simulink model "PfLoad"  (R2022a)
settings: Solver=ode14x  StartTime=0  StopTime=Sim.tend  FixedStep=0.000125  RelTol=4e-4
model workspace (MAT data in the model file):
  nr_load = Simulink.Parameter
  nr_load.Value = 2
  nr_load.DataType = 'int8'
  nr_load.Complexity = 'real'
  nr_load.Dimensions = [1 1]
values from neighbouring files (symbols this model uses):
  ControlSampleTime = 1/8000    (= 0.000125)    [sim3run_390.m]
  FB_area1_downlim = 49.5    [prm3var_390.m]
  FB_area1_uplim = 49.8    [prm3var_390.m]
  FB_area2_downlim = 49.2    [prm3var_390.m]
  FB_area2_uplim = 49.5    [prm3var_390.m]
  TVint = 0.05    [prm3var_390.m]
undefined symbols (not defined in the file or in its folder): DiscIntNeverNeededParam, General, parameterset, prm_load, pu_vsm, UFLS
libraries: simulink x2
settings Model: ParameterArgumentNames=nr_load  Creator=e2n052  LastModifiedBy=uk062294
settings DataIOCC: SaveOutput=off  SaveTime=off  ReturnWorkspaceOutputs=off
settings DebuggingCC: UnconnectedInputMsg=warning  UnconnectedOutputMsg=warning  UnconnectedLineMsg=warning  ArithmeticOperatorsInVariantConditions=warning
settings SFSimCC: SimUseLocalCustomCode=off  CustomCodeUndefinedFunction=UseInterfaceOnly
settings RTWCC: RTWUseLocalCustomCode=off  DLArmComputeVersion=19.05

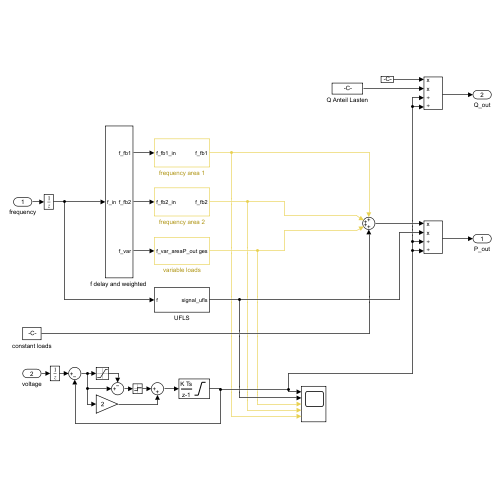
[thumbnail: Simulink's stored preview of the top-level diagram]
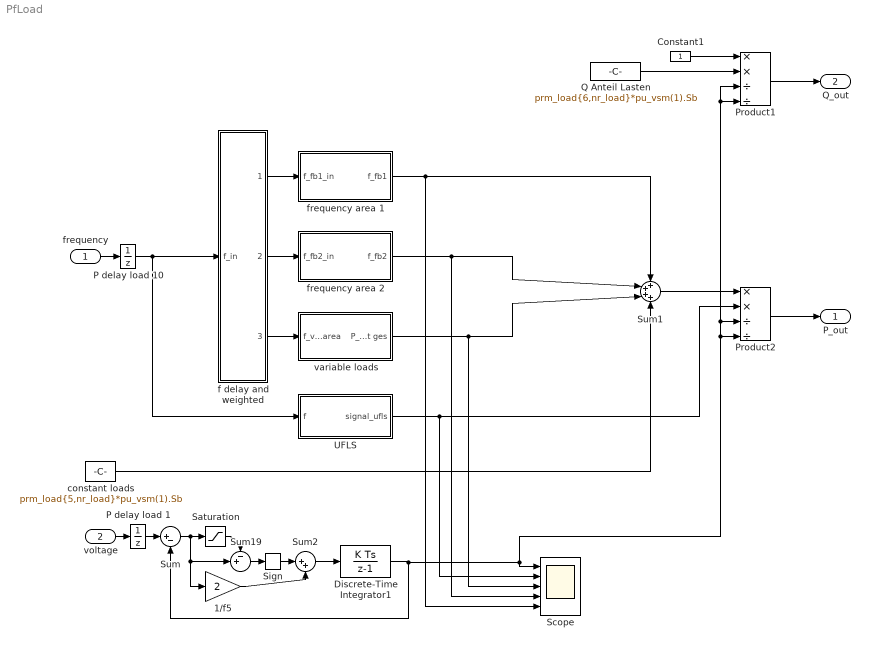
== system PfLoad ==
  frequency : Inport
  voltage : Inport  Port=2
  1/f5 : Gain  Gain=2
  Constant1 : Constant
  Discrete-Time Integrator1 : DiscreteIntegrator  gainval=1/TVint  InitialCondition=1  SampleTime=-1  LimitOutput=on  UpperSaturationLimit=1.15  LowerSaturationLimit=0.85  ICPrevOutput=DiscIntNeverNeededParam  ICPrevScaledInput=DiscIntNeverNeededParam
  P delay load 1 : UnitDelay  InitialCondition=General.Vnreg  SampleTime=-1  HasFrameUpgradeWarning=on
  P delay load 10 : UnitDelay  InitialCondition=General.fn  SampleTime=-1  HasFrameUpgradeWarning=on
  Product1 : Product  Inputs=**//
  Product2 : Product  Inputs=**//
  Q Anteil Lasten : Constant  Value=prm_load{6,nr_load}*pu_vsm(1).Sb
  Saturation : Saturate  UpperLimit=0.03  LowerLimit=-0.03
  Scope : Scope  NumInputPorts=5
  Sign : Signum
  Sum : Sum  Inputs=|+-
  Sum1 : Sum  Inputs=++++
  Sum19 : Sum  Inputs=-+|
  Sum2 : Sum  Inputs=|++
  UFLS : Subsystem
  constant loads : Constant  Value=prm_load{5,nr_load}*pu_vsm(1).Sb
  "f delay and weighted " : Subsystem
  frequency area 1 : Subsystem
  frequency area 2 : Subsystem
  variable loads : Subsystem
  P_out : Outport  OutDataTypeStr=double  PortDimensions=1
  Q_out : Outport  Port=2  OutDataTypeStr=double  PortDimensions=1
  wires:
  frequency area 1/1(f_fb1) -> Scope/5, Sum1/1
  frequency area 2/1(f_fb2) -> Scope/4, Sum1/2
  variable loads/1(P_out ges) -> Scope/3, Sum1/3
  constant loads/1 -> Sum1/4
  Sum1/1 -> Product2/1
  Constant1/1 -> Product1/1
  Q Anteil Lasten/1 -> Product1/2
  frequency/1 -> P delay load 10/1
  UFLS/1(signal_ufls) -> Scope/2, Product2/2
  "f delay and weighted "/1(f_fb1) -> frequency area 1/1(f_fb1_in)
  "f delay and weighted "/2(f_fb2) -> frequency area 2/1(f_fb2_in)
  "f delay and weighted "/3(f_var) -> variable loads/1(f_var_area)
  Sum/1 -> Sum19/2, 1/f5/1, Saturation/1
  Discrete-Time Integrator1/1 -> Sum/2, Scope/1, Product2/4, Product2/3, Product1/4, Product1/3
  Product1/1 -> Q_out/1
  Product2/1 -> P_out/1
  P delay load 10/1 -> "f delay and weighted "/1(f_in), UFLS/1(f)
  voltage/1 -> P delay load 1/1
  P delay load 1/1 -> Sum/1
  Saturation/1 -> Sum19/1
  Sign/1 -> Sum2/1
  Sum19/1 -> Sign/1
  Sum2/1 -> Discrete-Time Integrator1/1
  1/f5/1 -> Sum2/2

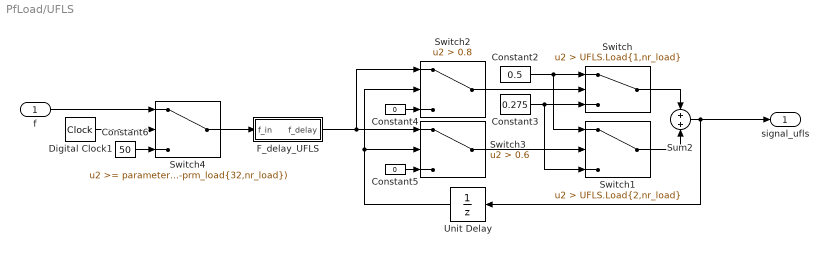
== system PfLoad/UFLS ==
  f : Inport
  Constant2 : Constant  Value=0.5
  Constant3 : Constant  Value=0.275
  Constant4 : Constant  Value=0
  Constant5 : Constant  Value=0
  Constant6 : Constant  Value=50
  Digital Clock1 : DigitalClock  SampleTime=ControlSampleTime
  F_delay_UFLS : Subsystem
  Sum2 : Sum  Inputs=+|+
  Switch : Switch  Criteria=u2 > Threshold  Threshold=UFLS.Load{1,nr_load}  SaturateOnIntegerOverflow=off  InputSameDT=off
  Switch1 : Switch  Criteria=u2 > Threshold  Threshold=UFLS.Load{2,nr_load}  SaturateOnIntegerOverflow=off  InputSameDT=off
  Switch2 : Switch  Criteria=u2 > Threshold  Threshold=0.8  SaturateOnIntegerOverflow=off  InputSameDT=off
  Switch3 : Switch  Criteria=u2 > Threshold  Threshold=0.6  SaturateOnIntegerOverflow=off  InputSameDT=off
  Switch4 : Switch  Threshold=parameterset.Event.IslandingTime-0.1+9e9*(1-prm_load{32,nr_load})  SaturateOnIntegerOverflow=off  InputSameDT=off
  Unit Delay : UnitDelay  InitialCondition=50  SampleTime=-1  HasFrameUpgradeWarning=on
  signal_ufls : Outport
  wires:
  Switch/1 -> Sum2/1
  Sum2/1 -> signal_ufls/1, Unit Delay/1
  Constant4/1 -> Switch2/3
  Constant3/1 -> Switch1/3, Switch/3
  Constant6/1 -> Switch4/3
  f/1 -> Switch4/1
  Switch3/1 -> Switch1/2
  Constant5/1 -> Switch3/3
  Unit Delay/1 -> Switch3/2, Switch2/2
  Constant2/1 -> Switch1/1, Switch/1
  Switch2/1 -> Switch/2
  Switch1/1 -> Sum2/2
  Switch4/1 -> F_delay_UFLS/1(f_in)
  F_delay_UFLS/1(f_delay) -> Switch2/1, Switch3/1
  Digital Clock1/1 -> Switch4/2

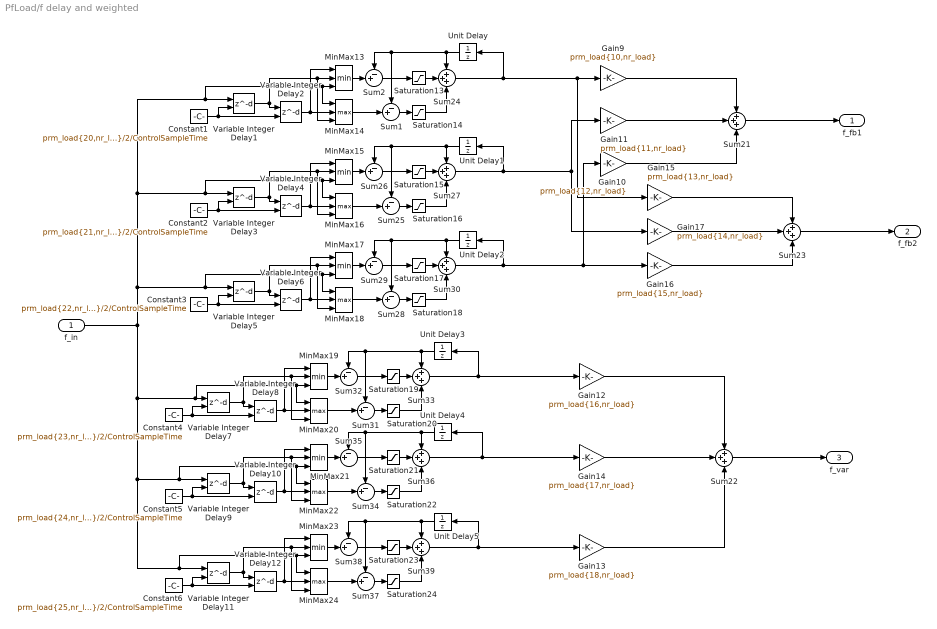
== system PfLoad/f delay and weighted  ==
  f_in : Inport
  Constant1 : Constant  Value=prm_load{20,nr_load}/2/ControlSampleTime
  Constant2 : Constant  Value=prm_load{21,nr_load}/2/ControlSampleTime
  Constant3 : Constant  Value=prm_load{22,nr_load}/2/ControlSampleTime
  Constant4 : Constant  Value=prm_load{23,nr_load}/2/ControlSampleTime
  Constant5 : Constant  Value=prm_load{24,nr_load}/2/ControlSampleTime
  Constant6 : Constant  Value=prm_load{25,nr_load}/2/ControlSampleTime
  Gain10 : Gain  Gain=prm_load{12,nr_load}
  Gain11 : Gain  Gain=prm_load{11,nr_load}
  Gain12 : Gain  Gain=prm_load{16,nr_load}
  Gain13 : Gain  Gain=prm_load{18,nr_load}
  Gain14 : Gain  Gain=prm_load{17,nr_load}
  Gain15 : Gain  Gain=prm_load{13,nr_load}
  Gain16 : Gain  Gain=prm_load{15,nr_load}
  Gain17 : Gain  Gain=prm_load{14,nr_load}
  Gain9 : Gain  Gain=prm_load{10,nr_load}
  MinMax{13,15,17,19,21,23} (6 alike) : MinMax  Inputs=3
  MinMax{14,16,18,20,22,24} (6 alike) : MinMax  Function=max  Inputs=3
  Saturation{13,15,17,19,21,23} (6 alike) : Saturate  UpperLimit=inf  LowerLimit=0
  Saturation{14,16,18,20,22,24} (6 alike) : Saturate  UpperLimit=0  LowerLimit=-inf
  Sum{1..2,25..26,28..29,31..32,34..35,37..38} (12 alike) : Sum  Inputs=-+|
  Sum{21..24,27,30,33,36,39} (9 alike) : Sum  Inputs=+++
  Unit Delay{,1..5} (6 alike) : UnitDelay  InitialCondition=General.fn  SampleTime=-1  HasFrameUpgradeWarning=on
  Variable Integer Delay{1..12} (12 alike) : Delay  DelayLengthSource=Input port  DelayLength=prm_load{21,nr_load}/2/ControlSampleTime  DelayLengthUpperLimit=5000
      settings: InputPortMap=u0,p1
  f_fb1 : Outport
  f_fb2 : Outport  Port=2
  f_var : Outport  Port=3
  wires:
  Gain14/1 -> Sum22/2
  Gain11/1 -> Sum21/2
  Gain10/1 -> Sum21/3
  Gain17/1 -> Sum23/2
  Gain15/1 -> Sum23/1
  Sum22/1 -> f_var/1
  Sum21/1 -> f_fb1/1
  Sum23/1 -> f_fb2/1
  Gain13/1 -> Sum22/3
  Gain16/1 -> Sum23/3
  Gain9/1 -> Sum21/1
  Gain12/1 -> Sum22/1
  Saturation14/1 -> Sum24/3
  Sum24/1 -> Unit Delay/1, Gain9/1, Gain15/1
  Sum1/1 -> Saturation14/1
  Unit Delay/1 -> Sum24/1, Sum2/1, Sum1/1
  Variable Integer Delay2/1 -> MinMax13/1, MinMax14/2
  Variable Integer Delay1/1 -> Variable Integer Delay2/1, MinMax14/3, MinMax13/2
  Constant1/1 -> Variable Integer Delay2/2, Variable Integer Delay1/2
  MinMax13/1 -> Sum2/2
  Sum2/1 -> Saturation13/1
  MinMax14/1 -> Sum1/2
  Saturation13/1 -> Sum24/2
  Saturation16/1 -> Sum27/3
  Sum25/1 -> Saturation16/1
  Unit Delay1/1 -> Sum27/1, Sum26/1, Sum25/1
  Variable Integer Delay4/1 -> MinMax15/1, MinMax16/2
  Variable Integer Delay3/1 -> Variable Integer Delay4/1, MinMax16/3, MinMax15/2
  Constant2/1 -> Variable Integer Delay4/2, Variable Integer Delay3/2
  MinMax15/1 -> Sum26/2
  Sum26/1 -> Saturation15/1
  MinMax16/1 -> Sum25/2
  Saturation15/1 -> Sum27/2
  Saturation18/1 -> Sum30/3
  Sum30/1 -> Unit Delay2/1, Gain10/1, Gain16/1
  Sum28/1 -> Saturation18/1
  Unit Delay2/1 -> Sum30/1, Sum29/1, Sum28/1
  Variable Integer Delay6/1 -> MinMax17/1, MinMax18/2
  Variable Integer Delay5/1 -> Variable Integer Delay6/1, MinMax18/3, MinMax17/2
  Constant3/1 -> Variable Integer Delay6/2, Variable Integer Delay5/2
  MinMax17/1 -> Sum29/2
  Sum29/1 -> Saturation17/1
  MinMax18/1 -> Sum28/2
  Saturation17/1 -> Sum30/2
  Saturation20/1 -> Sum33/3
  Sum31/1 -> Saturation20/1
  Unit Delay3/1 -> Sum33/1, Sum32/1, Sum31/1
  Variable Integer Delay8/1 -> MinMax19/1, MinMax20/2
  Variable Integer Delay7/1 -> Variable Integer Delay8/1, MinMax20/3, MinMax19/2
  Constant4/1 -> Variable Integer Delay8/2, Variable Integer Delay7/2
  MinMax19/1 -> Sum32/2
  Sum32/1 -> Saturation19/1
  MinMax20/1 -> Sum31/2
  Saturation19/1 -> Sum33/2
  Saturation22/1 -> Sum36/3
  Sum34/1 -> Saturation22/1
  Unit Delay4/1 -> Sum35/1, Sum34/1, Sum36/1
  Variable Integer Delay10/1 -> MinMax21/1, MinMax22/2
  Variable Integer Delay9/1 -> Variable Integer Delay10/1, MinMax22/3, MinMax21/2
  Constant5/1 -> Variable Integer Delay10/2, Variable Integer Delay9/2
  MinMax21/1 -> Sum35/2
  Sum35/1 -> Saturation21/1
  MinMax22/1 -> Sum34/2
  Saturation21/1 -> Sum36/2
  Saturation24/1 -> Sum39/3
  Sum37/1 -> Saturation24/1
  Unit Delay5/1 -> Sum39/1, Sum38/1, Sum37/1
  Variable Integer Delay12/1 -> MinMax23/1, MinMax24/2
  Variable Integer Delay11/1 -> Variable Integer Delay12/1, MinMax24/3, MinMax23/2
  f_in/1 -> MinMax24/1, MinMax23/3, Variable Integer Delay11/1, MinMax22/1, MinMax21/3, Variable Integer Delay9/1, MinMax20/1, MinMax19/3, Variable Integer Delay7/1, MinMax14/1, MinMax13/3, Variable Integer Delay1/1, MinMax16/1, MinMax15/3, Variable Integer Delay3/1, MinMax18/1, MinMax17/3, Variable Integer Delay5/1
  Constant6/1 -> Variable Integer Delay12/2, Variable Integer Delay11/2
  MinMax23/1 -> Sum38/2
  Sum38/1 -> Saturation23/1
  MinMax24/1 -> Sum37/2
  Saturation23/1 -> Sum39/2
  Sum27/1 -> Unit Delay1/1, Gain11/1, Gain17/1
  Sum33/1 -> Unit Delay3/1, Gain12/1
  Sum36/1 -> Unit Delay4/1, Gain14/1
  Sum39/1 -> Unit Delay5/1, Gain13/1

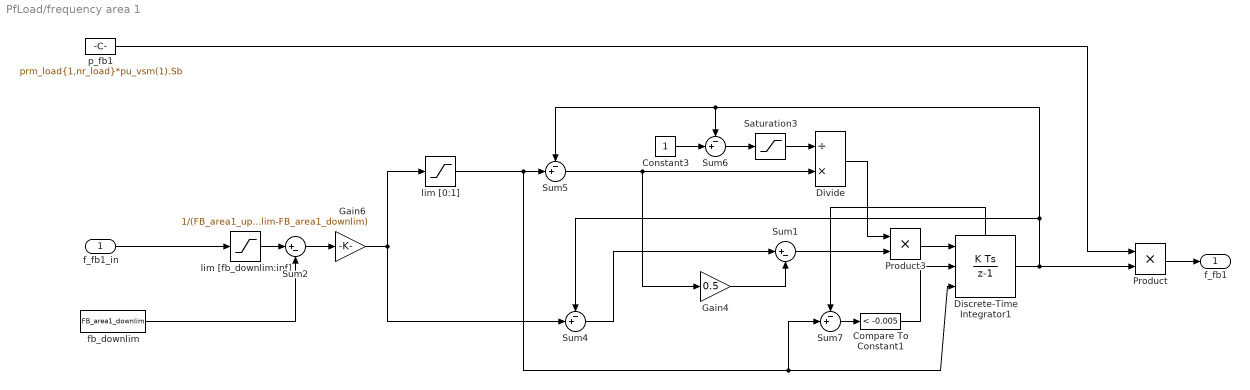
== system PfLoad/frequency area 1 ==
  f_fb1_in : Inport
  Compare To Constant1 : simulink/Logic and Bit Operations/Compare To Constant  relop=<  const=-0.005  OutDataTypeStr=boolean
  Constant3 : Constant
  Discrete-Time Integrator1 : DiscreteIntegrator  ExternalReset=level  InitialConditionSource=external  SampleTime=ControlSampleTime  LimitOutput=on  UpperSaturationLimit=1  LowerSaturationLimit=0  ShowStatePort=on  ICPrevOutput=DiscIntNeverNeededParam  ICPrevScaledInput=DiscIntNeverNeededParam
  Divide : Product  Inputs=/*
  Gain4 : Gain  Gain=0.5
  Gain6 : Gain  Gain=1/(FB_area1_uplim-FB_area1_downlim)
  Product : Product
  Product3 : Product
  Saturation3 : Saturate  UpperLimit=inf  LowerLimit=1e-6
  Sum1 : Sum  Inputs=|+-
  Sum2 : Sum  Inputs=|+-
  Sum{4..7} (4 alike) : Sum  Inputs=-+|
  fb_downlim : Constant  Value=FB_area1_downlim
  lim [0:1] : Saturate  UpperLimit=1  LowerLimit=0
  lim [fb_downlim:inf] : Saturate  UpperLimit=inf  LowerLimit=FB_area1_downlim
  p_fb1 : Constant  Value=prm_load{1,nr_load}*pu_vsm(1).Sb
  f_fb1 : Outport
  wires:
  Discrete-Time Integrator1/1 -> Sum5/1, Sum6/1, Sum4/1, Product/2
  Discrete-Time Integrator1/State -> Sum7/1
  Sum7/1 -> Compare To Constant1/1
  fb_downlim/1 -> Sum2/2
  f_fb1_in/1 -> lim [fb_downlim:inf]/1
  Compare To Constant1/1 -> Discrete-Time Integrator1/2
  Saturation3/1 -> Divide/1
  Divide/1 -> Product3/1
  Constant3/1 -> Sum6/2
  Gain6/1 -> Sum4/2, lim [0:1]/1
  Sum2/1 -> Gain6/1
  lim [fb_downlim:inf]/1 -> Sum2/1
  Sum4/1 -> Sum1/1
  Sum6/1 -> Saturation3/1
  Product3/1 -> Discrete-Time Integrator1/1
  Gain4/1 -> Sum1/2
  Sum5/1 -> Gain4/1, Divide/2
  Sum1/1 -> Product3/2
  lim [0:1]/1 -> Sum7/2, Discrete-Time Integrator1/3, Sum5/2
  Product/1 -> f_fb1/1
  p_fb1/1 -> Product/1

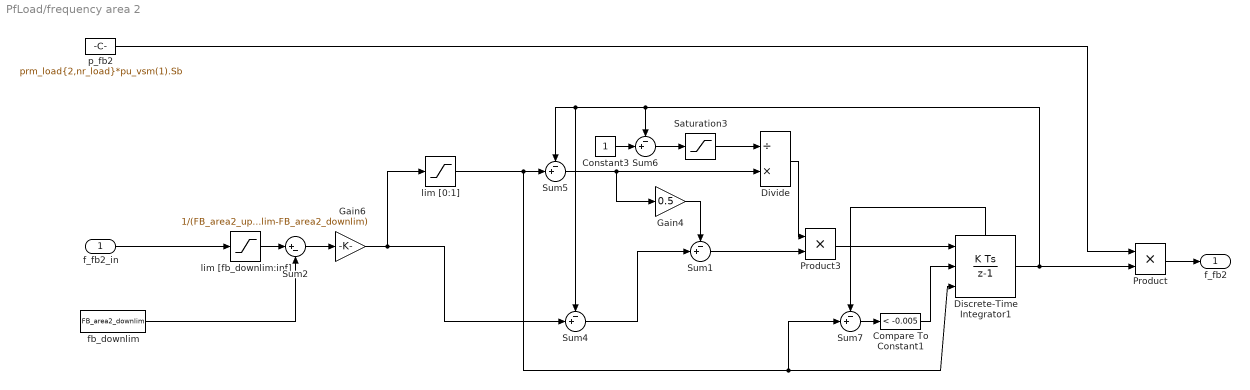
== system PfLoad/frequency area 2 ==
  f_fb2_in : Inport
  Compare To Constant1 : simulink/Logic and Bit Operations/Compare To Constant  relop=<  const=-0.005  OutDataTypeStr=boolean
  Constant3 : Constant
  Discrete-Time Integrator1 : DiscreteIntegrator  ExternalReset=level  InitialConditionSource=external  SampleTime=ControlSampleTime  LimitOutput=on  UpperSaturationLimit=1  LowerSaturationLimit=0  ShowStatePort=on  ICPrevOutput=DiscIntNeverNeededParam  ICPrevScaledInput=DiscIntNeverNeededParam
  Divide : Product  Inputs=/*
  Gain4 : Gain  Gain=0.5
  Gain6 : Gain  Gain=1/(FB_area2_uplim-FB_area2_downlim)
  Product : Product
  Product3 : Product
  Saturation3 : Saturate  UpperLimit=inf  LowerLimit=1e-6
  Sum{1,4..7} (5 alike) : Sum  Inputs=-+|
  Sum2 : Sum  Inputs=|+-
  fb_downlim : Constant  Value=FB_area2_downlim
  lim [0:1] : Saturate  UpperLimit=1  LowerLimit=0
  lim [fb_downlim:inf] : Saturate  UpperLimit=inf  LowerLimit=FB_area2_downlim
  p_fb2 : Constant  Value=prm_load{2,nr_load}*pu_vsm(1).Sb
  f_fb2 : Outport
  wires:
  Discrete-Time Integrator1/1 -> Sum4/1, Sum5/1, Sum6/1, Product/2
  Discrete-Time Integrator1/State -> Sum7/1
  Sum7/1 -> Compare To Constant1/1
  fb_downlim/1 -> Sum2/2
  f_fb2_in/1 -> lim [fb_downlim:inf]/1
  Compare To Constant1/1 -> Discrete-Time Integrator1/2
  Saturation3/1 -> Divide/1
  Divide/1 -> Product3/1
  Constant3/1 -> Sum6/2
  Gain6/1 -> Sum4/2, lim [0:1]/1
  Sum2/1 -> Gain6/1
  lim [fb_downlim:inf]/1 -> Sum2/1
  Sum4/1 -> Sum1/2
  Sum6/1 -> Saturation3/1
  Product3/1 -> Discrete-Time Integrator1/1
  Gain4/1 -> Sum1/1
  Sum5/1 -> Divide/2, Gain4/1
  Sum1/1 -> Product3/2
  lim [0:1]/1 -> Sum7/2, Discrete-Time Integrator1/3, Sum5/2
  Product/1 -> f_fb2/1
  p_fb2/1 -> Product/1

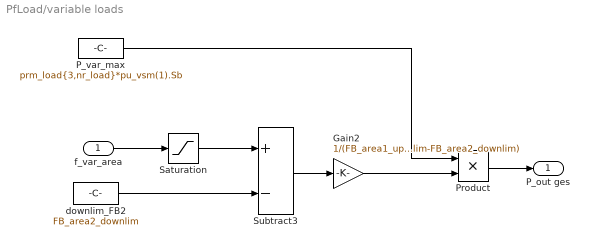
== system PfLoad/variable loads ==
  f_var_area : Inport
  Gain2 : Gain  Gain=1/(FB_area1_uplim-FB_area2_downlim)
  P_var_max : Constant  Value=prm_load{3,nr_load}*pu_vsm(1).Sb
  Product : Product
  Saturation : Saturate  UpperLimit=FB_area1_uplim  LowerLimit=FB_area2_downlim
  Subtract3 : Sum  Inputs=+-
  downlim_FB2 : Constant  Value=FB_area2_downlim
  P_out ges : Outport
  wires:
  Gain2/1 -> Product/2
  Subtract3/1 -> Gain2/1
  downlim_FB2/1 -> Subtract3/2
  f_var_area/1 -> Saturation/1
  P_var_max/1 -> Product/1
  Product/1 -> P_out ges/1
  Saturation/1 -> Subtract3/1

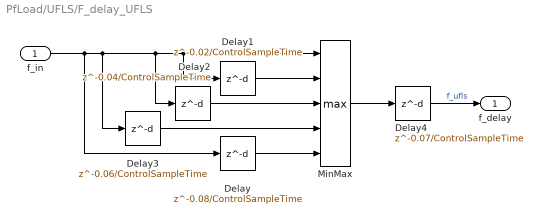
== system PfLoad/UFLS/F_delay_UFLS ==
  f_in : Inport
  Delay : Delay  DelayLength=0.08/ControlSampleTime
  Delay1 : Delay  DelayLength=0.02/ControlSampleTime  InitialCondition=General.fn
  Delay2 : Delay  DelayLength=0.04/ControlSampleTime  InitialCondition=General.fn
  Delay3 : Delay  DelayLength=0.06/ControlSampleTime  InitialCondition=General.fn
  Delay4 : Delay  DelayLength=0.07/ControlSampleTime  InitialCondition=General.fn
  MinMax : MinMax  Function=max  Inputs=5
  f_delay : Outport
  wires:
  MinMax/1 -> Delay4/1
  f_in/1 -> Delay/1, Delay3/1, Delay2/1, Delay1/1, MinMax/1
  Delay2/1 -> MinMax/3
  Delay1/1 -> MinMax/2
  Delay3/1 -> MinMax/4
  Delay/1 -> MinMax/5
  Delay4/1 -> f_delay/1  "f_ufls"
